simulink model "Refined_Model_38"  (R2020b)
settings: Solver=FixedStepAuto  StartTime=0.0  StopTime=500  FixedStep=0.1  RelTol=1e-3
values from neighbouring files (symbols this model uses):
  CovDist = RoadProfile(:,4)    [ICE_Val.m]
  Cx = VehicleDefine(7,3)    [BEV_Basictest.m]    (also in GPS_val.m; ICEBEV_Script.m; ICEBEV_Script_VECTO.m; ICE_Script.m)
  Dist = 1:length(MaxSpeedProfile)    [GPS_val.m]    (also in ICE_Script.m; ICE_Val.m = [1:CovDist(end)])
  DynRolRad = VehicleDefine(5,3)    [BEV_Basictest.m]    (also in GPS_val.m; ICEBEV_Script.m; ICEBEV_Script_VECTO.m; ICE_Script.m)
  EngineRpm = round(IntpTorCur(:,1))    [GPS_val.m]    (also in ICEBEV_Script.m; ICEBEV_Script_VECTO.m; ICE_Script.m; ICE_Script_SSVal.m)
  etaClutch = VehicleDefine(23,3)    [GPS_val.m]    (also in ICEBEV_Script.m; ICEBEV_Script_VECTO.m; ICE_Script.m; ICE_Script_SSVal.m)
  FCTableVal = FCMap(2:end,2:end)    [GPS_val.m]    (also in ICEBEV_Script.m; ICEBEV_Script_VECTO.m; ICE_Script.m; ICE_Script_SSVal.m)
  FDR = VehicleDefine(20,3)    [BEV_Basictest.m]    (also in GPS_val.m = VehicleDefine(22,3); ICEBEV_Script.m = VehicleDefine(22,3); ICEBEV_Script_VECTO.m = VehicleDefine(22,3); ICE_Script.m = VehicleDefine(22,3))
  Fr = VehicleDefine(13,3)    [BEV_Basictest.m]    (also in GPS_val.m; ICEBEV_Script.m; ICEBEV_Script_VECTO.m; ICE_Script.m)
  g = VehicleDefine(14,3)    [BEV_Basictest.m]    (also in GPS_val.m; ICEBEV_Script.m; ICEBEV_Script_VECTO.m; ICE_Script.m)
  GNo = GBXDefine(:,1)    [GPS_val.m]    (also in ICEBEV_Script.m; ICEBEV_Script_VECTO.m; ICE_Script.m; ICE_Script_SSVal.m)
  GRa = GBXDefine(:,2)    [GPS_val.m]    (also in ICEBEV_Script.m; ICEBEV_Script_VECTO.m; ICE_Script.m; ICE_Script_SSVal.m)
  InitVel = VehicleDefine(21,3)    [BEV_Basictest.m]    (also in GPS_val.m = VehicleDefine(24,3); ICEBEV_Script.m = VehicleDefine(24,3); ICEBEV_Script_VECTO.m = VehicleDefine(24,3); ICE_Script.m = VehicleDefine(24,3))
  IntpSlope = round(IntpSlope,1)    [GPS_val.m]    (also in ICE_Script.m; ICE_Val.m = A)
  Je = VehicleDefine(25,3)    [GPS_val.m]    (also in ICEBEV_Script.m; ICEBEV_Script_VECTO.m; ICE_Script.m; ICE_Script_SSVal.m)
  Jk = VehicleDefine(15,3)    [BEV_Basictest.m]    (also in GPS_val.m; ICEBEV_Script.m; ICEBEV_Script_VECTO.m; ICE_Script.m)
  Jm = VehicleDefine(16,3)    [GPS_val.m]    (also in ICEBEV_Script.m; ICEBEV_Script_VECTO.m; ICE_Script.m; ICE_Script_SSVal.m)
  MaxAcc = 1    [BEV_Basictest.m]    (also in GPS_val.m; ICEBEV_Script.m; ICEBEV_Script_VECTO.m; ICE_Script.m)
  MaxDec = 1    [BEV_Basictest.m]    (also in GPS_val.m; ICEBEV_Script.m; ICEBEV_Script_VECTO.m; ICE_Script.m)
  MaxSpeedProfile = FMSP    [GPS_val.m]    (also in ICE_Script.m; ICE_Val.m = repelem(SegSPLatinmps,SegLeninm))
  MaxTorValThrot = max(ThrotTableVal,[],2)    [GPS_val.m]    (also in ICEBEV_Script.m; ICEBEV_Script_VECTO.m; ICE_Script.m; ICE_Script_SSVal.m)
  Me = VehicleDefine(10,3)    [BEV_Basictest.m]    (also in GPS_val.m; ICEBEV_Script.m; ICEBEV_Script_VECTO.m; ICE_Script.m)
  MotoringTor = IntpTorCur(:,3)    [GPS_val.m]    (also in ICEBEV_Script.m; ICEBEV_Script_VECTO.m; ICE_Script.m; ICE_Script_SSVal.m)
  Mt = VehicleDefine(12,3)    [BEV_Basictest.m]    (also in GPS_val.m; ICEBEV_Script.m; ICEBEV_Script_VECTO.m; ICE_Script.m)
  Mtot = Mv+Me+Mt    [BEV_Basictest.m]    (also in GPS_val.m; ICEBEV_Script.m; ICEBEV_Script_VECTO.m; ICE_Script.m)
  Mv = VehicleDefine(9,3)    [BEV_Basictest.m]    (also in GPS_val.m; ICEBEV_Script.m; ICEBEV_Script_VECTO.m; ICE_Script.m)
  NoSteps = round(Dist(end))    [GPS_val.m]    (also in ICE_Script.m; ICE_Val.m = 3002)
  NoWhlFA = VehicleDefine(2,3)    [BEV_Basictest.m]    (also in GPS_val.m; ICE_Script.m; ICE_Val.m; ICE_Val_new.m)
  NoWhlRA = VehicleDefine(4,3)    [BEV_Basictest.m]    (also in GPS_val.m; ICE_Script.m; ICE_Val.m; ICE_Val_new.m)
  rho = VehicleDefine(6,3)    [BEV_Basictest.m]    (also in GPS_val.m; ICEBEV_Script.m; ICEBEV_Script_VECTO.m; ICE_Script.m)
  RpmBrkPnt = ThrottleMap(1,:)    [GPS_val.m]    (also in ICEBEV_Script.m; ICEBEV_Script_VECTO.m; ICE_Script.m; ICE_Script_SSVal.m)
  s = divisors(length(MaxSpeedProfile))    [GPS_val.m]    (also in ICEBEV_Script.m = round(FLoadTor); ICEBEV_Script_VECTO.m = round(FLoadTor); ICE_Script.m = round(FLoadTor); ICE_Script_SSVal.m = round(FLoadTor))
  SegNo = RoadProfile(:,1)    [ICE_Val.m]
  SegSPLatinmps = (sqrt(aMaxLat*g*CurRadinm))    [GPS_val.m]    (also in ICE_Script.m; ICE_Val.m)
  Sx = VehicleDefine(8,3)    [BEV_Basictest.m]    (also in GPS_val.m; ICEBEV_Script.m; ICEBEV_Script_VECTO.m; ICE_Script.m)
  ThrotPos = ThrotPos'    [GPS_val.m]    (also in ICEBEV_Script.m; ICEBEV_Script_VECTO.m; ICE_Script.m; ICE_Script_SSVal.m)
  ThrotTableVal = ThrottleMap(2:end,2:end)    [GPS_val.m]    (also in ICEBEV_Script.m; ICEBEV_Script_VECTO.m; ICE_Script.m; ICE_Script_SSVal.m)
undefined symbols (not defined in the file or in its folder): G1Inprpm, GInprpm, GInpTor, GTorLoss, MaxSpinG, MaxWhlTorinG, Stoptimes
libraries: simulink x3, autolibshared x1
settings Model: Creator=Kshitij  LastModifiedBy=Kshitij
settings DebuggingCC: AlgebraicLoopMsg=none

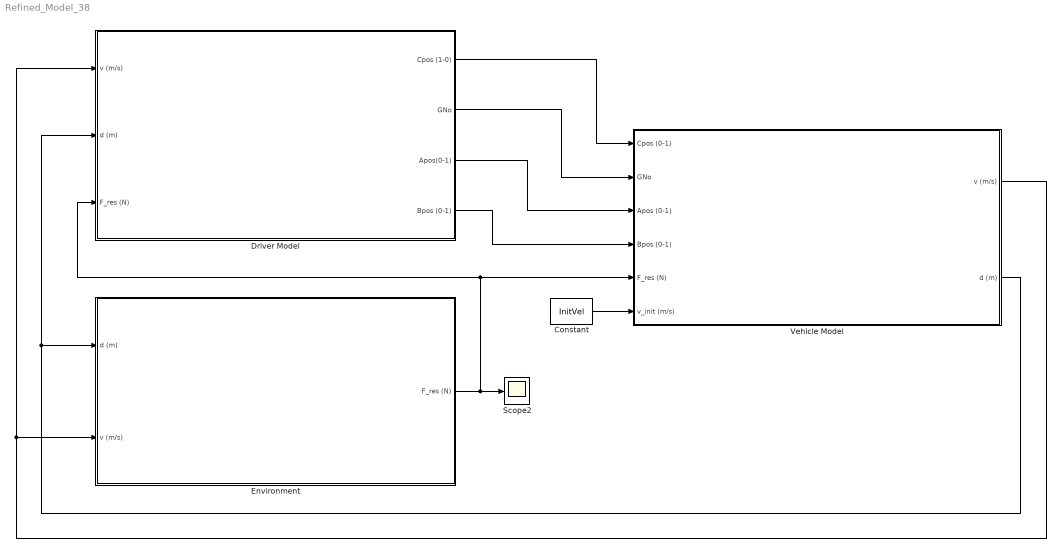
== system Refined_Model_38 ==
  Constant : Constant  Value=InitVel
  Driver Model : Subsystem
  Environment : Subsystem
  Scope2 : Scope
  Vehicle Model : Subsystem
  wires:
  Environment/1(F_res (N)) -> Driver Model/3(F_res (N)), Vehicle Model/5(F_res (N)), Scope2/1
  Vehicle Model/2(d (m)) -> Driver Model/2(d (m)), Environment/1(d (m))
  Vehicle Model/1(v (m/s)) -> Driver Model/1(v (m/s)), Environment/2(v (m/s))
  Constant/1 -> Vehicle Model/6(v_init (m/s))
  Driver Model/1(Cpos (1-0)) -> Vehicle Model/1(Cpos (0-1))
  Driver Model/2(GNo) -> Vehicle Model/2(GNo)
  Driver Model/3(Apos(0-1)) -> Vehicle Model/3(Apos (0-1))
  Driver Model/4(Bpos (0-1)) -> Vehicle Model/4(Bpos (0-1))

== system Refined_Model_38/Driver Model ==
  v (m/s) : Inport
  d (m) : Inport  Port=2
  F_res (N) : Inport  Port=3
  Acc/Dec Control : Subsystem
  Driver Throttle : Subsystem
  Gear and Clutch Definition : Subsystem
  Scope1 : Scope  NumInputPorts=2
  Cpos (1-0) : Outport
  GNo : Outport  Port=2
  Apos(0-1) : Outport  Port=3
  Bpos (0-1) : Outport  Port=4
  wires:
  Acc/Dec Control/2(Bpos (0-1)) -> Bpos (0-1)/1, Scope1/2  "Bpos (0-1)"
  d (m)/1 -> Acc/Dec Control/2(d (m))
  Gear and Clutch Definition/1(Cpos) -> Cpos (1-0)/1
  v (m/s)/1 -> Gear and Clutch Definition/2(v (m/s)), Acc/Dec Control/1(v (m/s))
  Gear and Clutch Definition/2(GNo) -> GNo/1, Driver Throttle/1(GNo)
  Driver Throttle/2(Apos (0-1)) -> Scope1/1, Apos(0-1)/1  "Apos(0-1)"
  Driver Throttle/1(T_w_req (Nm)) -> Gear and Clutch Definition/1(T_w_req (Nm))  "T_w_req (Nm)"
  F_res (N)/1 -> Driver Throttle/2(F_res (N))
  Acc/Dec Control/1(Apos(m/s^2)) -> Driver Throttle/3(Apos(m/s^2))

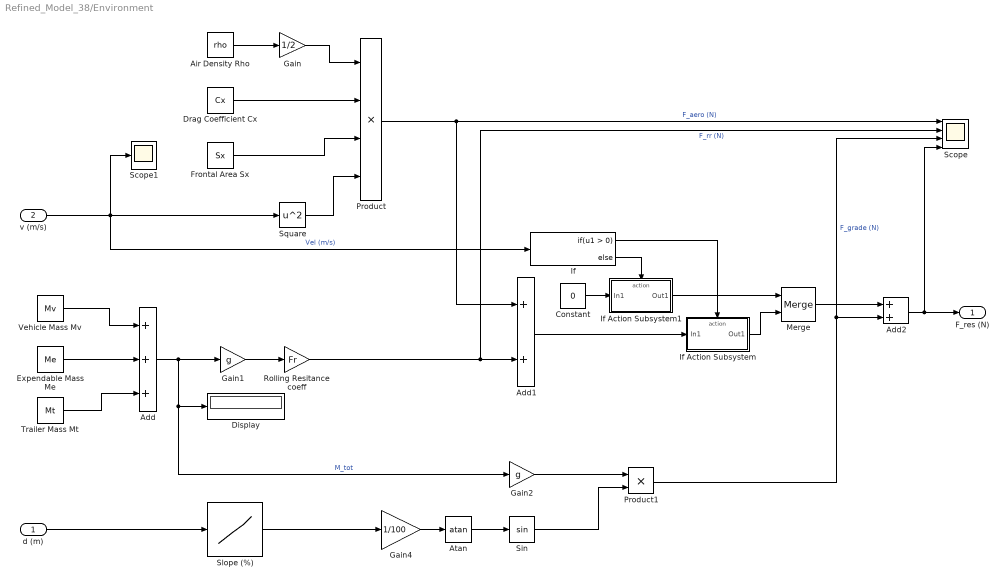
== system Refined_Model_38/Environment ==
  d (m) : Inport
  v (m/s) : Inport  Port=2
  Add : Sum  Inputs=+++
  Add1 : Sum
  Add2 : Sum
  Air Density Rho : Constant  Value=rho
  Atan : Trigonometry  Operator=atan
  Constant : Constant  Value=0
  Display : Display
  Drag Coefficient Cx : Constant  Value=Cx
  Expendable Mass Me : Constant  Value=Me
  Frontal Area Sx : Constant  Value=Sx
  Gain : Gain  Gain=1/2
  Gain1 : Gain  Gain=g
  Gain2 : Gain  Gain=g
  Gain4 : Gain  Gain=1/100
  If : If
  If Action Subsystem : Subsystem  TreatAsAtomicUnit=on
  If Action Subsystem1 : Subsystem  TreatAsAtomicUnit=on
  Merge : Merge
  Product : Product  Inputs=4
  Product1 : Product
  Rolling Resitance coeff : Gain  Gain=Fr
  Scope : Scope  NumInputPorts=4
  Scope1 : Scope
  Sin : Trigonometry
  Slope (%) : Lookup_n-D  NumberOfTableDimensions=1  BreakpointsForDimension1=Dist  Table=IntpSlope  InternalRulePriority=Speed  RndMeth=Simplest  InputSameDT=on
  Square : Math  Operator=square  SaturateOnIntegerOverflow=on
  Trailer Mass Mt : Constant  Value=Mt
  Vehicle Mass Mv : Constant  Value=Mv
  F_res (N) : Outport
  wires:
  Expendable Mass Me/1 -> Add/2
  Add/1 -> Display/1, Gain2/1, Gain1/1  "M_tot"
  Gain/1 -> Product/1
  Sin/1 -> Product1/2
  Product1/1 -> Scope/3, Add2/2  "F_grade (N)"
  Air Density Rho/1 -> Gain/1
  Drag Coefficient Cx/1 -> Product/2
  v (m/s)/1 -> Scope1/1, Square/1, If/1  "Vel (m/s)"
  d (m)/1 -> Slope (%)/1
  Gain2/1 -> Product1/1
  Trailer Mass Mt/1 -> Add/3
  Rolling Resitance coeff/1 -> Scope/2, Add1/2  "F_rr (N)"
  Square/1 -> Product/4
  Gain1/1 -> Rolling Resitance coeff/1
  Vehicle Mass Mv/1 -> Add/1
  Product/1 -> Scope/1, Add1/1  "F_aero (N)"
  Frontal Area Sx/1 -> Product/3
  If/1 -> If Action Subsystem/Action
  If/2 -> If Action Subsystem1/Action
  If Action Subsystem1/1(Out1) -> Merge/1
  Add1/1 -> If Action Subsystem/1(In1)
  If Action Subsystem/1(Out1) -> Merge/2
  Constant/1 -> If Action Subsystem1/1(In1)
  Merge/1 -> Add2/1
  Add2/1 -> F_res (N)/1, Scope/4
  Slope (%)/1 -> Gain4/1
  Atan/1 -> Sin/1
  Gain4/1 -> Atan/1

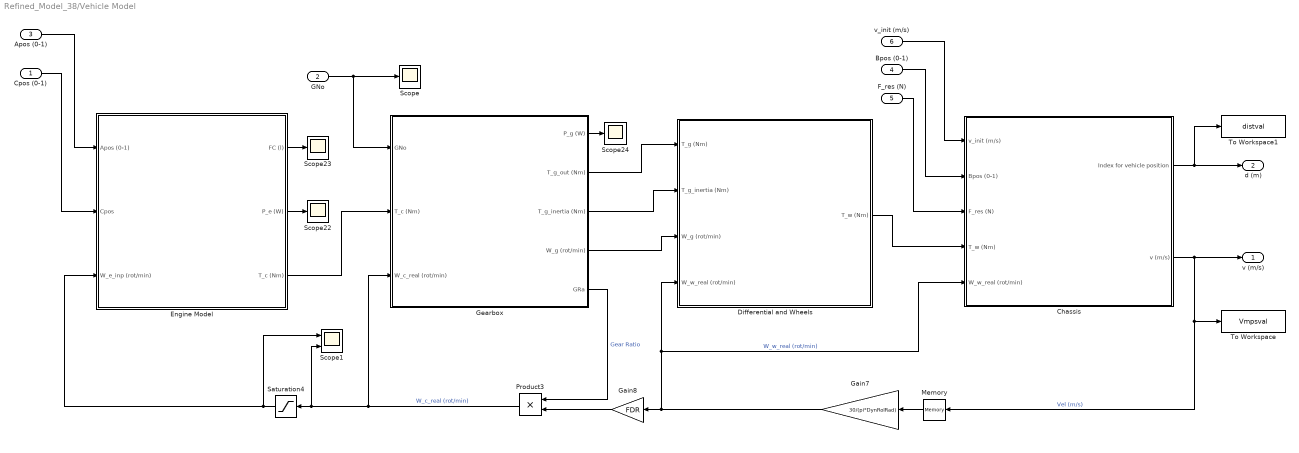
== system Refined_Model_38/Vehicle Model ==
  Cpos (0-1) : Inport
  GNo : Inport  Port=2
  Apos (0-1) : Inport  Port=3
  Bpos (0-1) : Inport  Port=4
  F_res (N) : Inport  Port=5
  v_init (m/s) : Inport  Port=6
  Chassis : Subsystem
  Differential and Wheels : Subsystem
  Engine Model : Subsystem
  Gain7 : Gain  Gain=30/(pi*DynRolRad)
  Gain8 : Gain  Gain=FDR
  Gearbox : Subsystem
  Memory : Memory
  Product3 : Product
  Saturation4 : Saturate  UpperLimit=max(EngineRpm)  LowerLimit=min(EngineRpm)
  Scope{,22..24} (4 alike) : Scope
  Scope1 : Scope  NumInputPorts=2
  To Workspace : ToWorkspace  VariableName=Vmpsval  SaveFormat=Timeseries  SampleTime=-1
  To Workspace1 : ToWorkspace  VariableName=distval  SaveFormat=Timeseries  SampleTime=-1
  v (m/s) : Outport
  d (m) : Outport  Port=2
  wires:
  Gearbox/2(T_g_out (Nm)) -> Differential and Wheels/1(T_g (Nm))
  Gearbox/4(W_g (rot/min)) -> Differential and Wheels/3(W_g (rot/min))
  Gearbox/3(T_g_inertia (Nm)) -> Differential and Wheels/2(T_g_inertia (Nm))
  Chassis/1(Index for vehicle position) -> To Workspace1/1, d (m)/1
  Bpos (0-1)/1 -> Chassis/2(Bpos (0-1))
  v_init (m/s)/1 -> Chassis/1(v_init (m/s))
  Differential and Wheels/1(T_w (Nm)) -> Chassis/4(T_w (Nm))
  F_res (N)/1 -> Chassis/3(F_res (N))
  Gearbox/1(P_g (W)) -> Scope24/1
  Engine Model/3(T_c (Nm)) -> Gearbox/2(T_c (Nm))
  Apos (0-1)/1 -> Engine Model/1(Apos (0-1))
  Engine Model/2(P_e (W)) -> Scope22/1
  Engine Model/1(FC (l)) -> Scope23/1
  GNo/1 -> Gearbox/1(GNo), Scope/1
  Chassis/2(v (m/s)) -> v (m/s)/1, Memory/1, To Workspace/1  "Vel (m/s)"
  Gearbox/5(GRa) -> Product3/1  "Gear Ratio"
  Gain8/1 -> Product3/2
  Gain7/1 -> Gain8/1, Chassis/5(W_w_real (rot/min)), Differential and Wheels/4(W_w_real (rot/min))  "W_w_real (rot/min)"
  Cpos (0-1)/1 -> Engine Model/2(Cpos)
  Product3/1 -> Scope1/2, Saturation4/1, Gearbox/3(W_c_real (rot/min))  "W_c_real (rot/min)"
  Saturation4/1 -> Scope1/1, Engine Model/3(W_e_inp (rot/min))
  Memory/1 -> Gain7/1

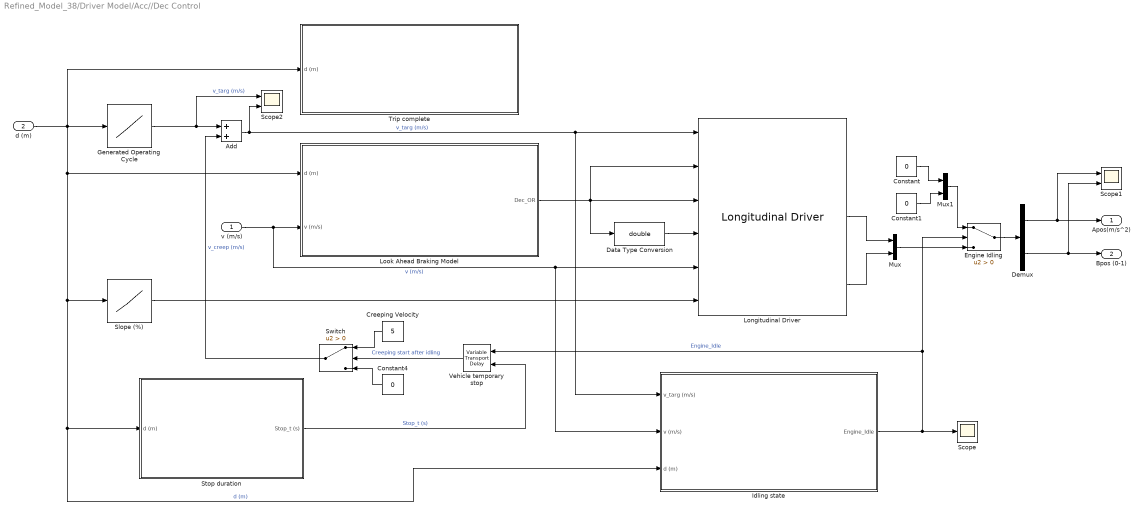
== system Refined_Model_38/Driver Model/Acc//Dec Control ==
  v (m/s) : Inport
  d (m) : Inport  Port=2
  Add : Sum
  Constant : Constant  Value=0
  Constant1 : Constant  Value=0
  Constant4 : Constant  Value=0
  Creeping Velocity : Constant  Value=5
  Data Type Conversion : DataTypeConversion  OutDataTypeStr=double
  Demux : Demux  Outputs=2
  Engine Idling : Switch  Criteria=u2 > Threshold
  Generated Operating Cycle : Lookup_n-D  NumberOfTableDimensions=1  BreakpointsForDimension1=Dist  BreakpointsForDimension2=G1Inprpm  Table=MaxSpeedProfile  InterpMethod=Linear Lagrange  InternalRulePriority=Speed  RndMeth=Simplest  InputSameDT=on
  Idling state : Subsystem
  Longitudinal Driver : autolibshared/Longitudinal Driver  extAccelOvr=off  extDecelOvr=on  extAccelHld=off  extDecelHld=off  extAccelZero=on  extDecelZero=off  cntrlType=PI  shftType=None  velUnits=m/s  gearOut=off  Kp=150  Ki=1000  Kff=0  Kg=0  VehVelVec=[0 100]  KffVec=[.1 .1]  KpVec=[10 10]  KiVec=[5 5]  KgVec=[0 0]  m=1500  Kpt=3000  tau=.1  L=2  aR=200  bR=2.5  cR=.5  g=9.81  vnom=100  Kaw=0  tauerr=0  tauPt=2  GearInit=0  tShift=.1  pdlVec=[0.1 0.4 0.5 0.9]  upShftTbl=[-1 12.9375 26.4375 39.9375 51.18749999999999 62.4375 72.84375 83.25;-1 16.3125 29.8125 43.3125 54.5624 65.8125 76.78125 87.75;-1 19.6875 33.1875 46.68749999999999 57.9375 69.1875 80.71875 92.25;-1 33 52.5 77.25 100.5 138.75 161.875 185]  dwnShftTbl=[1 9.5625 23.0625 36.5625 47.8125 59.0625 68.90625 78.75;1 12.9375 26.4375 39.9375 51.18749999999999 62.4375 72.84375 83.25;1 16.3125 29.8125 43.3125 54.562499 65.8125 76.78125 87.75;1 19.6875 33.1875 46.68749999999999 57.9375 69.1875 80.71875 92.25]  tClutch=.5  tRev=.5  tPark=120  aMode=1  UpGearVec="[0  1  2  3  4  5  6  7]"  DownGearVec="[1  2  3  4  5  6  7  8]"
      settings: SourceProductBaseCode=PW,MT,UV,VE,VP
  Look Ahead Braking Model : Subsystem
  Mux : Mux  Inputs=2
  Mux1 : Mux  Inputs=2
  Scope : Scope
  Scope1 : Scope  NumInputPorts=2
  Scope2 : Scope  NumInputPorts=2
  Slope (%) : Lookup_n-D  NumberOfTableDimensions=1  BreakpointsForDimension1=Dist  Table=IntpSlope  InternalRulePriority=Speed  RndMeth=Simplest  InputSameDT=on
  Stop duration : Subsystem
  Switch : Switch  Criteria=u2 > Threshold
  Trip complete : Subsystem
  Vehicle temporary stop : VariableTransportDelay  VariableDelayType=Variable transport delay  MaximumDelay=10
  Apos(m/s^2) : Outport
  Bpos (0-1) : Outport  Port=2
  wires:
  Add/1 -> Scope2/2, Idling state/1(v_targ (m/s)), Longitudinal Driver/1  "v_targ (m/s)"
  Slope (%)/1 -> Longitudinal Driver/6
  Longitudinal Driver/2 -> Mux/1
  Look Ahead Braking Model/1(Dec_OR) -> Longitudinal Driver/2, Longitudinal Driver/3, Data Type Conversion/1
  Demux/1 -> Scope1/1, Apos(m/s^2)/1
  Demux/2 -> Scope1/2, Bpos (0-1)/1
  Constant/1 -> Mux1/1
  Mux/1 -> Engine Idling/3
  Constant1/1 -> Mux1/2
  Mux1/1 -> Engine Idling/1
  Engine Idling/1 -> Demux/1
  d (m)/1 -> Idling state/3(d (m)), Stop duration/1(d (m)), Slope (%)/1, Look Ahead Braking Model/1(d (m)), Trip complete/1(d (m)), Generated Operating Cycle/1  "d (m)"
  v (m/s)/1 -> Longitudinal Driver/5, Idling state/2(v (m/s)), Look Ahead Braking Model/2(v (m/s))  "v (m/s)"
  Generated Operating Cycle/1 -> Scope2/1, Add/1  "v_targ (m/s)"
  Vehicle temporary stop/1 -> Switch/2  "Creeping start after idling"
  Switch/1 -> Add/2  "v_creep (m/s)"
  Constant4/1 -> Switch/3
  Creeping Velocity/1 -> Switch/1
  Idling state/1(Engine_Idle) -> Scope/1, Engine Idling/2, Vehicle temporary stop/1  "Engine_Idle"
  Stop duration/1(Stop_t (s)) -> Vehicle temporary stop/2  "Stop_t (s)"
  Data Type Conversion/1 -> Longitudinal Driver/4
  Longitudinal Driver/3 -> Mux/2

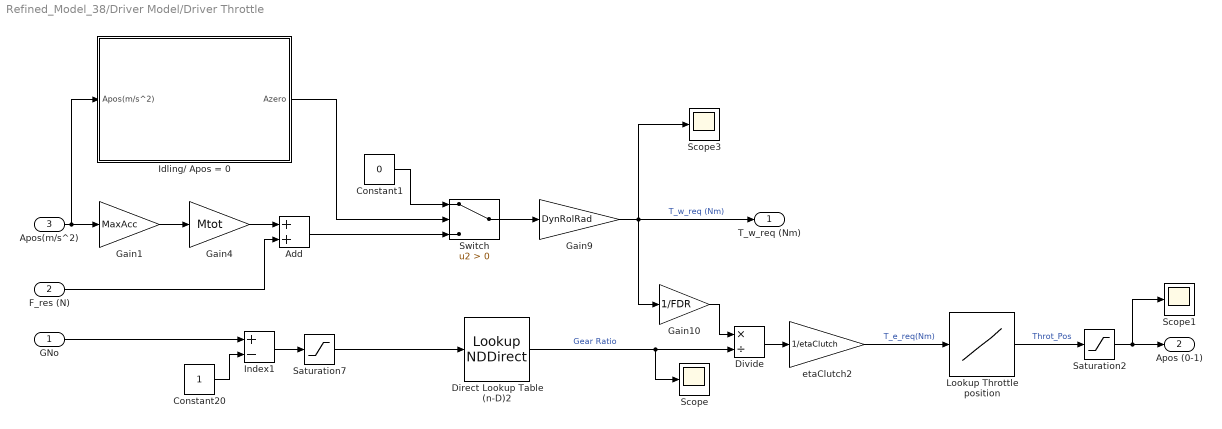
== system Refined_Model_38/Driver Model/Driver Throttle ==
  GNo : Inport
  F_res (N) : Inport  Port=2
  Apos(m/s^2) : Inport  Port=3
  Add : Sum
  Constant1 : Constant  Value=0
  Constant20 : Constant
  Direct Lookup Table (n-D)2 : LookupNDDirect  NumberOfTableDimensions=1  Table=GRa
  Divide : Product  Inputs=*/
  Gain1 : Gain  Gain=MaxAcc
  Gain10 : Gain  Gain=1/FDR
  Gain4 : Gain  Gain=Mtot
  Gain9 : Gain  Gain=DynRolRad
  Idling/ Apos = 0 : Subsystem
  Index1 : Sum  Inputs=+-
  Lookup Throttle position : Lookup_n-D  NumberOfTableDimensions=1  BreakpointsForDimension1=MaxTorValThrot  Table=ThrotPos  InternalRulePriority=Speed  RndMeth=Simplest  InputSameDT=on
  Saturation2 : Saturate  UpperLimit=1  LowerLimit=0
  Saturation7 : Saturate  UpperLimit=inf  LowerLimit=0
  Scope : Scope
  Scope1 : Scope
  Scope3 : Scope
  Switch : Switch  Criteria=u2 > Threshold
  etaClutch2 : Gain  Gain=1/etaClutch
  T_w_req (Nm) : Outport
  Apos (0-1) : Outport  Port=2
  wires:
  etaClutch2/1 -> Lookup Throttle position/1  "T_e_req(Nm)"
  Add/1 -> Switch/3
  Gain9/1 -> Scope3/1, T_w_req (Nm)/1, Gain10/1  "T_w_req (Nm)"
  Gain10/1 -> Divide/1
  Gain4/1 -> Add/1
  Divide/1 -> etaClutch2/1
  F_res (N)/1 -> Add/2
  Lookup Throttle position/1 -> Saturation2/1  "Throt_Pos"
  Saturation2/1 -> Apos (0-1)/1, Scope1/1
  Apos(m/s^2)/1 -> Idling/ Apos = 0/1(Apos(m/s^2)), Gain1/1
  Gain1/1 -> Gain4/1
  Constant20/1 -> Index1/2
  GNo/1 -> Index1/1
  Index1/1 -> Saturation7/1
  Saturation7/1 -> Direct Lookup Table (n-D)2/1
  Direct Lookup Table (n-D)2/1 -> Scope/1, Divide/2  "Gear Ratio"
  Switch/1 -> Gain9/1
  Constant1/1 -> Switch/1
  Idling/ Apos = 0/1(Azero) -> Switch/2

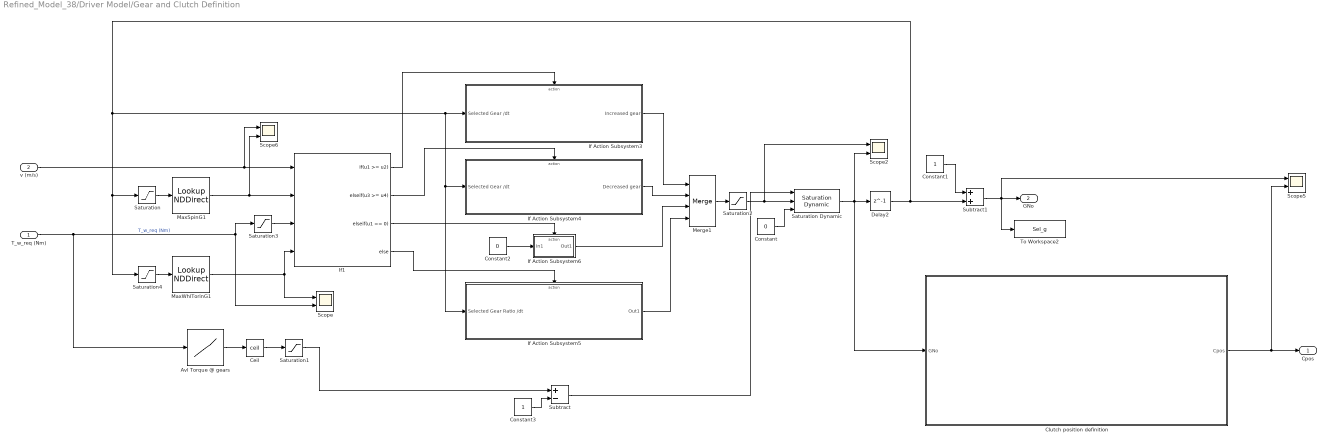
== system Refined_Model_38/Driver Model/Gear and Clutch Definition ==
  T_w_req (Nm) : Inport
  v (m/s) : Inport  Port=2
  Avl Torque @ gears : Lookup_n-D  NumberOfTableDimensions=1  BreakpointsForDimension1=flip(MaxWhlTorinG)  Table=flip(GNo)  InternalRulePriority=Speed  RndMeth=Simplest  InputSameDT=on
  Ceil : Rounding  Operator=ceil
  Clutch position definition : Subsystem
  Constant : Constant  Value=0
  Constant1 : Constant
  Constant2 : Constant  Value=0
  Constant3 : Constant
  Delay2 : Delay  DelayLength=1
  If Action Subsystem3 : Subsystem  TreatAsAtomicUnit=on
  If Action Subsystem4 : Subsystem  TreatAsAtomicUnit=on
  If Action Subsystem5 : Subsystem  TreatAsAtomicUnit=on
  If Action Subsystem6 : Subsystem  TreatAsAtomicUnit=on
  If1 : If  NumInputs=4  IfExpression=u1 >= u2  ElseIfExpressions=u3 >= u4,u1 == 0
  MaxSpinG1 : LookupNDDirect  NumberOfTableDimensions=1  Table=MaxSpinG
  MaxWhlTorinG1 : LookupNDDirect  NumberOfTableDimensions=1  Table=MaxWhlTorinG
  Merge1 : Merge  Inputs=4
  Saturation : Saturate  UpperLimit=inf  LowerLimit=0
  Saturation Dynamic : simulink/Discontinuities/Saturation Dynamic  OutMin=[]  OutMax=[]  OutDataTypeStr=Inherit: Same as second input  OutDataType=fixdt(1, 16)  OutScaling=2^-10  DoSatur=off
  Saturation1 : Saturate  UpperLimit=max(GNo)  LowerLimit=0
  Saturation2 : Saturate  UpperLimit=max(GNo)-1  LowerLimit=0
  Saturation3 : Saturate  UpperLimit=inf  LowerLimit=0
  Saturation4 : Saturate  UpperLimit=inf  LowerLimit=0
  Scope{,2,5..6} (4 alike) : Scope  NumInputPorts=2
  Subtract : Sum  Inputs=+-
  Subtract1 : Sum
  To Workspace2 : ToWorkspace  VariableName=Sel_g  SaveFormat=Timeseries  SampleTime=-1
  Cpos : Outport
  GNo : Outport  Port=2
  wires:
  Clutch position definition/1(Cpos) -> Scope5/2, Cpos/1
  If1/2 -> If Action Subsystem4/Action
  If Action Subsystem4/1(Decreased gear) -> Merge1/2
  If1/4 -> If Action Subsystem5/Action
  If Action Subsystem3/1(Increased gear) -> Merge1/1
  MaxSpinG1/1 -> Scope6/2, If1/2
  If Action Subsystem5/1(Out1) -> Merge1/4
  MaxWhlTorinG1/1 -> Scope/1, If1/4
  If1/1 -> If Action Subsystem3/Action
  Saturation3/1 -> If1/3
  T_w_req (Nm)/1 -> Saturation3/1, Scope/2, Avl Torque @ gears/1  "T_w_req (Nm)"
  Constant1/1 -> Subtract1/1
  Saturation/1 -> MaxSpinG1/1
  Saturation4/1 -> MaxWhlTorinG1/1
  Delay2/1 -> Subtract1/2, If Action Subsystem3/1(Selected Gear /dt), If Action Subsystem5/1(Selected Gear Ratio /dt), If Action Subsystem4/1(Selected Gear /dt), Saturation/1, Saturation4/1
  Subtract1/1 -> Scope5/1, GNo/1, To Workspace2/1
  v (m/s)/1 -> Scope6/1, If1/1
  If1/3 -> If Action Subsystem6/Action
  Constant2/1 -> If Action Subsystem6/1(In1)
  If Action Subsystem6/1(Out1) -> Merge1/3
  Merge1/1 -> Saturation2/1
  Avl Torque @ gears/1 -> Ceil/1
  Ceil/1 -> Saturation1/1
  Saturation Dynamic/1 -> Scope2/2, Clutch position definition/1(GNo), Delay2/1
  Subtract/1 -> Saturation Dynamic/1
  Constant3/1 -> Subtract/2
  Saturation1/1 -> Subtract/1
  Saturation2/1 -> Scope2/1, Saturation Dynamic/2
  Constant/1 -> Saturation Dynamic/3

== system Refined_Model_38/Environment/If Action Subsystem ==
  In1 : Inport
  Action Port : ActionPort  ActionPortLabel=if(u1 > 0)
  Out1 : Outport
  wires:
  In1/1 -> Out1/1

== system Refined_Model_38/Environment/If Action Subsystem1 ==
  In1 : Inport
  Action Port : ActionPort  ActionPortLabel=else
  Out1 : Outport
  wires:
  In1/1 -> Out1/1

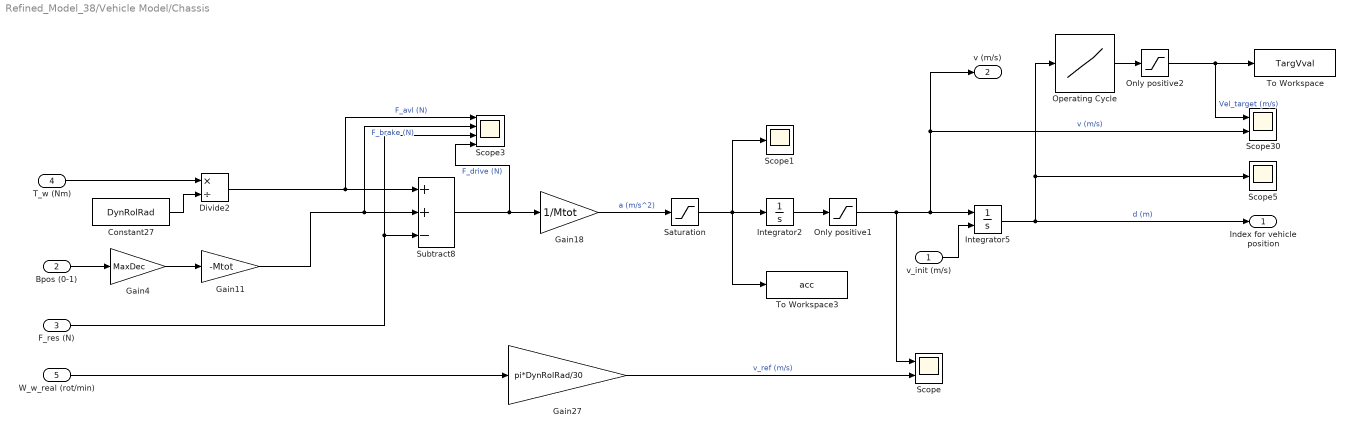
== system Refined_Model_38/Vehicle Model/Chassis ==
  v_init (m/s) : Inport
  Bpos (0-1) : Inport  Port=2
  F_res (N) : Inport  Port=3
  T_w (Nm) : Inport  Port=4
  W_w_real (rot/min) : Inport  Port=5
  Constant27 : Constant  Value=DynRolRad
  Divide2 : Product  Inputs=*/
  Gain11 : Gain  Gain=-Mtot
  Gain18 : Gain  Gain=1/Mtot
  Gain27 : Gain  Gain=pi*DynRolRad/30
  Gain4 : Gain  Gain=MaxDec
  Integrator2 : Integrator  ContinuousStateAttributes='acceleration'
  Integrator5 : Integrator  InitialConditionSource=external  ContinuousStateAttributes='velocity'
  Only positive1 : Saturate  UpperLimit=inf  LowerLimit=0
  Only positive2 : Saturate  UpperLimit=inf  LowerLimit=0
  Operating Cycle : Lookup_n-D  NumberOfTableDimensions=1  BreakpointsForDimension1=Dist  BreakpointsForDimension2=G1Inprpm  Table=MaxSpeedProfile  InterpMethod=Linear Lagrange  InternalRulePriority=Speed  RndMeth=Simplest  InputSameDT=on
  Saturation : Saturate  UpperLimit=MaxAcc  LowerLimit=-(MaxDec)
  Scope : Scope  NumInputPorts=2
  Scope1 : Scope
  Scope3 : Scope  NumInputPorts=4
  Scope30 : Scope  NumInputPorts=2
  Scope5 : Scope
  Subtract8 : Sum  Inputs=++-
  To Workspace : ToWorkspace  VariableName=TargVval  SaveFormat=Timeseries  SampleTime=-1
  To Workspace3 : ToWorkspace  VariableName=acc  SaveFormat=Timeseries  SampleTime=-1
  Index for vehicle position : Outport
  v (m/s) : Outport  Port=2
  wires:
  Constant27/1 -> Divide2/2
  Subtract8/1 -> Scope3/4, Gain18/1  "F_drive (N)"
  Divide2/1 -> Subtract8/1, Scope3/1  "F_avl (N)"
  Integrator5/1 -> Index for vehicle position/1, Scope5/1, Operating Cycle/1  "d (m)"
  Integrator2/1 -> Only positive1/1
  T_w (Nm)/1 -> Divide2/1
  Gain11/1 -> Subtract8/2, Scope3/2  "F_brake (N)"
  Only positive1/1 -> Scope/1, v (m/s)/1, Scope30/2, Integrator5/1  "v (m/s)"
  v_init (m/s)/1 -> Integrator5/2
  Gain27/1 -> Scope/2  "v_ref (m/s)"
  Operating Cycle/1 -> Only positive2/1
  Gain18/1 -> Saturation/1  "a (m/s^2)"
  W_w_real (rot/min)/1 -> Gain27/1
  Bpos (0-1)/1 -> Gain4/1
  Gain4/1 -> Gain11/1
  F_res (N)/1 -> Subtract8/3, Scope3/3
  Saturation/1 -> Integrator2/1, To Workspace3/1, Scope1/1
  Only positive2/1 -> To Workspace/1, Scope30/1  "Vel_target (m/s)"

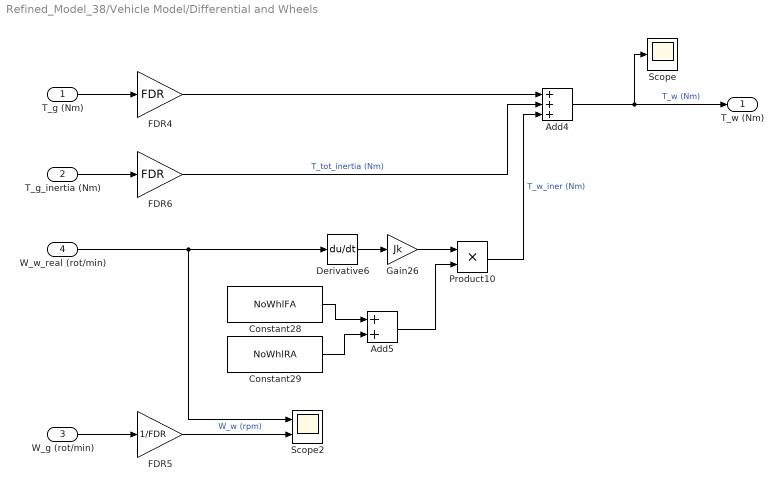
== system Refined_Model_38/Vehicle Model/Differential and Wheels ==
  T_g (Nm) : Inport
  T_g_inertia (Nm) : Inport  Port=2
  W_g (rot/min) : Inport  Port=3
  W_w_real (rot/min) : Inport  Port=4
  Add4 : Sum  Inputs=+++
  Add5 : Sum
  Constant28 : Constant  Value=NoWhlFA
  Constant29 : Constant  Value=NoWhlRA
  Derivative6 : Derivative
  FDR4 : Gain  Gain=FDR
  FDR5 : Gain  Gain=1/FDR
  FDR6 : Gain  Gain=FDR
  Gain26 : Gain  Gain=Jk
  Product10 : Product
  Scope : Scope
  Scope2 : Scope  NumInputPorts=2
  T_w (Nm) : Outport
  wires:
  Product10/1 -> Add4/3  "T_w_iner (Nm)"
  Derivative6/1 -> Gain26/1
  Add5/1 -> Product10/2
  Constant29/1 -> Add5/2
  FDR6/1 -> Add4/2  "T_tot_inertia (Nm)"
  Constant28/1 -> Add5/1
  FDR4/1 -> Add4/1
  FDR5/1 -> Scope2/2  "W_w (rpm)"
  Gain26/1 -> Product10/1
  T_g_inertia (Nm)/1 -> FDR6/1
  Add4/1 -> Scope/1, T_w (Nm)/1  "T_w (Nm)"
  T_g (Nm)/1 -> FDR4/1
  W_g (rot/min)/1 -> FDR5/1
  W_w_real (rot/min)/1 -> Scope2/1, Derivative6/1

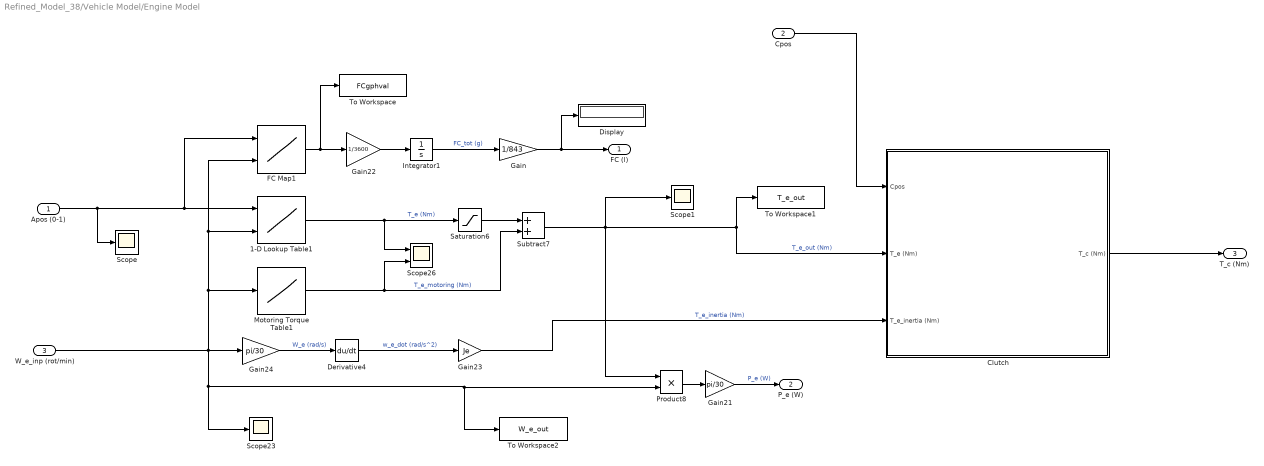
== system Refined_Model_38/Vehicle Model/Engine Model ==
  Apos (0-1) : Inport
  Cpos : Inport  Port=2
  W_e_inp (rot/min) : Inport  Port=3
  1-D Lookup Table1 : Lookup_n-D  BreakpointsForDimension1=ThrotPos  BreakpointsForDimension2=RpmBrkPnt  Table=ThrotTableVal  InternalRulePriority=Speed  RndMeth=Simplest  InputSameDT=on
      settings: InputPortMap=u0,u1
  Clutch : Subsystem
  Derivative4 : Derivative
  Display : Display
  FC Map1 : Lookup_n-D  BreakpointsForDimension1=ThrotPos  BreakpointsForDimension2=RpmBrkPnt  Table=FCTableVal  InternalRulePriority=Speed  RndMeth=Simplest  InputSameDT=on
      settings: InputPortMap=u0,u1
  Gain : Gain  Gain=1/843
  Gain21 : Gain  Gain=pi/30
  Gain22 : Gain  Gain=1/3600
  Gain23 : Gain  Gain=Je
  Gain24 : Gain  Gain=pi/30
  Integrator1 : Integrator
  Motoring Torque Table1 : Lookup_n-D  NumberOfTableDimensions=1  BreakpointsForDimension1=EngineRpm  BreakpointsForDimension2=G1Inprpm  Table=MotoringTor  InterpMethod=Linear Lagrange  InternalRulePriority=Speed  RndMeth=Simplest  InputSameDT=on
  Product8 : Product
  Saturation6 : Saturate  UpperLimit=inf  LowerLimit=0
  Scope : Scope
  Scope1 : Scope
  Scope23 : Scope
  Scope26 : Scope  NumInputPorts=2
  Subtract7 : Sum
  To Workspace : ToWorkspace  VariableName=FCgphval  SaveFormat=Timeseries  SampleTime=-1
  To Workspace1 : ToWorkspace  VariableName=T_e_out  SaveFormat=Timeseries  SampleTime=-1
  To Workspace2 : ToWorkspace  VariableName=W_e_out  SaveFormat=Timeseries  SampleTime=-1
  FC (l) : Outport
  P_e (W) : Outport  Port=2
  T_c (Nm) : Outport  Port=3
  wires:
  Motoring Torque Table1/1 -> Subtract7/2, Scope26/2  "T_e_motoring (Nm)"
  Integrator1/1 -> Gain/1  "FC_tot (g)"
  Derivative4/1 -> Gain23/1  "w_e_dot (rad/s^2)"
  W_e_inp (rot/min)/1 -> Scope23/1, To Workspace2/1, Product8/2, FC Map1/2, 1-D Lookup Table1/2, Motoring Torque Table1/1, Gain24/1
  Product8/1 -> Gain21/1
  Apos (0-1)/1 -> FC Map1/1, 1-D Lookup Table1/1, Scope/1
  1-D Lookup Table1/1 -> Saturation6/1, Scope26/1  "T_e (Nm)"
  Gain24/1 -> Derivative4/1  "W_e (rad/s)"
  Gain23/1 -> Clutch/3(T_e_inertia (Nm))  "T_e_inertia (Nm)"
  Gain21/1 -> P_e (W)/1  "P_e (W)"
  Gain22/1 -> Integrator1/1
  Subtract7/1 -> To Workspace1/1, Clutch/2(T_e (Nm)), Scope1/1, Product8/1  "T_e_out (Nm)"
  FC Map1/1 -> To Workspace/1, Gain22/1
  Saturation6/1 -> Subtract7/1
  Clutch/1(T_c (Nm)) -> T_c (Nm)/1
  Cpos/1 -> Clutch/1(Cpos)
  Gain/1 -> Display/1, FC (l)/1

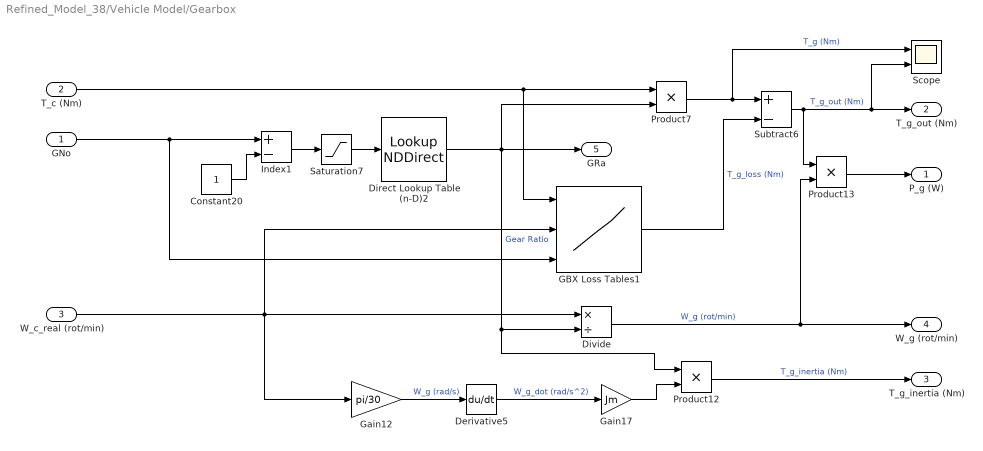
== system Refined_Model_38/Vehicle Model/Gearbox ==
  GNo : Inport
  T_c (Nm) : Inport  Port=2
  W_c_real (rot/min) : Inport  Port=3
  Constant20 : Constant
  Derivative5 : Derivative
  Direct Lookup Table (n-D)2 : LookupNDDirect  NumberOfTableDimensions=1  Table=GRa
  Divide : Product  Inputs=*/
  GBX Loss Tables1 : Lookup_n-D  NumberOfTableDimensions=3  BreakpointsForDimension1=GInpTor  BreakpointsForDimension2=GInprpm  BreakpointsForDimension3=GNo  Table=GTorLoss  InterpMethod=Linear Lagrange  InternalRulePriority=Speed  RndMeth=Simplest  InputSameDT=on
      settings: InputPortMap=u0,u1,u2
  Gain12 : Gain  Gain=pi/30
  Gain17 : Gain  Gain=Jm
  Index1 : Sum  Inputs=+-
  Product12 : Product
  Product13 : Product
  Product7 : Product
  Saturation7 : Saturate  UpperLimit=inf  LowerLimit=0
  Scope : Scope  NumInputPorts=2
  Subtract6 : Sum  Inputs=+-
  P_g (W) : Outport
  T_g_out (Nm) : Outport  Port=2
  T_g_inertia (Nm) : Outport  Port=3
  W_g (rot/min) : Outport  Port=4
  GRa : Outport  Port=5
  wires:
  Product12/1 -> T_g_inertia (Nm)/1  "T_g_inertia (Nm)"
  GNo/1 -> GBX Loss Tables1/3, Index1/1
  Gain17/1 -> Product12/2
  T_c (Nm)/1 -> GBX Loss Tables1/1, Product7/1
  Product7/1 -> Scope/1, Subtract6/1  "T_g (Nm)"
  Divide/1 -> W_g (rot/min)/1, Product13/2  "W_g (rot/min)"
  Subtract6/1 -> Scope/2, T_g_out (Nm)/1, Product13/1  "T_g_out (Nm)"
  Derivative5/1 -> Gain17/1  "W_g_dot (rad/s^2)"
  Direct Lookup Table (n-D)2/1 -> Product7/2, GRa/1, Product12/1, Divide/2  "Gear Ratio"
  Saturation7/1 -> Direct Lookup Table (n-D)2/1
  Gain12/1 -> Derivative5/1  "W_g (rad/s)"
  Constant20/1 -> Index1/2
  GBX Loss Tables1/1 -> Subtract6/2  "T_g_loss (Nm)"
  Index1/1 -> Saturation7/1
  Product13/1 -> P_g (W)/1
  W_c_real (rot/min)/1 -> GBX Loss Tables1/2, Gain12/1, Divide/1

== system Refined_Model_38/Driver Model/Acc//Dec Control/Idling state ==
  v_targ (m/s) : Inport
  v (m/s) : Inport  Port=2
  d (m) : Inport  Port=3
  Constant2 : Constant
  Constant3 : Constant  Value=0
  Delay : Delay  DelayLength=1
  Idling at stop point : If  NumInputs=3  IfExpression=u1 == 0 & u2 < 0 & u3 > 10
  If Action Subsystem : Subsystem  TreatAsAtomicUnit=on
  If Action Subsystem1 : Subsystem  TreatAsAtomicUnit=on
  Merge : Merge
  Subtract : Sum  Inputs=+-
  Engine_Idle : Outport
  wires:
  Subtract/1 -> Idling at stop point/2
  d (m)/1 -> Idling at stop point/3
  Constant2/1 -> If Action Subsystem/1(In1)
  If Action Subsystem/1(Out1) -> Merge/1
  Merge/1 -> Delay/1
  Idling at stop point/1 -> If Action Subsystem/Action
  Constant3/1 -> If Action Subsystem1/1(In1)
  v (m/s)/1 -> Subtract/2, Idling at stop point/1
  Idling at stop point/2 -> If Action Subsystem1/Action
  If Action Subsystem1/1(Out1) -> Merge/2
  Delay/1 -> Engine_Idle/1
  v_targ (m/s)/1 -> Subtract/1

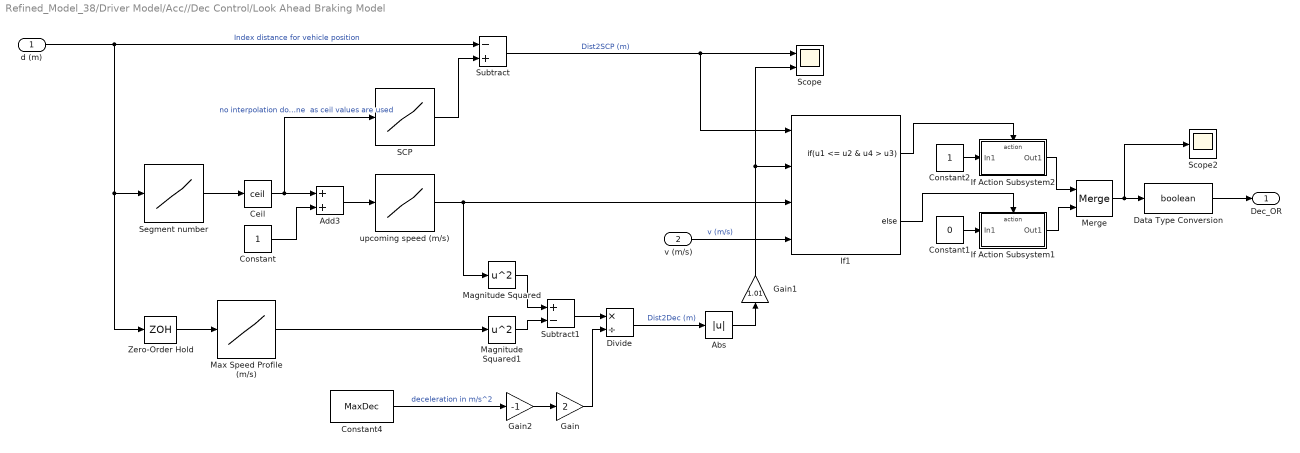
== system Refined_Model_38/Driver Model/Acc//Dec Control/Look Ahead Braking Model ==
  d (m) : Inport
  v (m/s) : Inport  Port=2
  Abs : Abs
  Add3 : Sum
  Ceil : Rounding  Operator=ceil
  Constant : Constant
  Constant1 : Constant  Value=0
  Constant2 : Constant
  Constant4 : Constant  Value=MaxDec
  Data Type Conversion : DataTypeConversion  OutDataTypeStr=boolean
  Divide : Product  Inputs=*/
  Gain : Gain  Gain=2
  Gain1 : Gain  Gain=1.01
  Gain2 : Gain  Gain=-1
  If Action Subsystem1 : Subsystem  TreatAsAtomicUnit=on
  If Action Subsystem2 : Subsystem  TreatAsAtomicUnit=on
  If1 : If  NumInputs=4  IfExpression=u1 <= u2 & u4 > u3
  Magnitude Squared : Math  Operator=square  SaturateOnIntegerOverflow=on
  Magnitude Squared1 : Math  Operator=square  SaturateOnIntegerOverflow=on
  Max Speed Profile (m/s) : Lookup_n-D  NumberOfTableDimensions=1  BreakpointsForDimension1=Dist  BreakpointsForDimension2=G1Inprpm  Table=MaxSpeedProfile  InterpMethod=Linear Lagrange  InternalRulePriority=Speed  RndMeth=Simplest  InputSameDT=on
  Merge : Merge
  SCP : Lookup_n-D  NumberOfTableDimensions=1  BreakpointsForDimension1=SegNo  BreakpointsForDimension2=G1Inprpm  Table=CovDist  InterpMethod=Linear Lagrange  InternalRulePriority=Speed  RndMeth=Simplest  InputSameDT=on
  Scope : Scope  NumInputPorts=2
  Scope2 : Scope
  Segment number : Lookup_n-D  NumberOfTableDimensions=1  BreakpointsForDimension1=CovDist  BreakpointsForDimension2=G1Inprpm  Table=SegNo  InterpMethod=Linear Lagrange  InternalRulePriority=Speed  RndMeth=Simplest  InputSameDT=on
  Subtract : Sum  Inputs=-+
  Subtract1 : Sum  Inputs=+-
  Zero-Order Hold : ZeroOrderHold  SampleTime=-1
  upcoming speed (m/s) : Lookup_n-D  NumberOfTableDimensions=1  BreakpointsForDimension1=SegNo  BreakpointsForDimension2=G1Inprpm  Table=SegSPLatinmps  InterpMethod=Linear Lagrange  InternalRulePriority=Speed  RndMeth=Simplest  InputSameDT=on
  Dec_OR : Outport
  wires:
  Add3/1 -> upcoming speed (m/s)/1
  Ceil/1 -> Add3/1, SCP/1  "no interpolation done  as ceil values are used"
  SCP/1 -> Subtract/2
  Constant/1 -> Add3/2
  Subtract/1 -> If1/1, Scope/1  "Dist2SCP (m)"
  Segment number/1 -> Ceil/1
  Magnitude Squared/1 -> Subtract1/1
  Constant4/1 -> Gain2/1  "deceleration in m/s^2"
  Divide/1 -> Abs/1  "Dist2Dec (m)"
  Constant1/1 -> If Action Subsystem1/1(In1)
  Constant2/1 -> If Action Subsystem2/1(In1)
  If1/1 -> If Action Subsystem2/Action
  If Action Subsystem2/1(Out1) -> Merge/1
  Magnitude Squared1/1 -> Subtract1/2
  Merge/1 -> Data Type Conversion/1, Scope2/1
  Data Type Conversion/1 -> Dec_OR/1
  Max Speed Profile (m/s)/1 -> Magnitude Squared1/1
  d (m)/1 -> Subtract/1, Zero-Order Hold/1, Segment number/1  "Index distance for vehicle position"
  Subtract1/1 -> Divide/1
  Gain2/1 -> Gain/1
  Gain/1 -> Divide/2
  If1/2 -> If Action Subsystem1/Action
  Zero-Order Hold/1 -> Max Speed Profile (m/s)/1
  If Action Subsystem1/1(Out1) -> Merge/2
  v (m/s)/1 -> If1/4  "v (m/s)"
  upcoming speed (m/s)/1 -> If1/3, Magnitude Squared/1
  Abs/1 -> Gain1/1
  Gain1/1 -> Scope/2, If1/2

== system Refined_Model_38/Driver Model/Acc//Dec Control/Stop duration ==
  d (m) : Inport
  1-D Lookup Table : Lookup_n-D  NumberOfTableDimensions=1  BreakpointsForDimension1=Stoptimes(:,1)  Table=1:length(Stoptimes)  InternalRulePriority=Speed  RndMeth=Simplest  InputSameDT=on
  Ceil : Rounding  Operator=ceil
  Constant2 : Constant
  Direct Lookup Table (n-D) : LookupNDDirect  NumberOfTableDimensions=1  Table=Stoptimes(:,2)
  Scope : Scope
  Subtract1 : Sum  Inputs=+-
  Stop_t (s) : Outport
  wires:
  1-D Lookup Table/1 -> Ceil/1
  d (m)/1 -> 1-D Lookup Table/1
  Subtract1/1 -> Direct Lookup Table (n-D)/1
  Direct Lookup Table (n-D)/1 -> Stop_t (s)/1, Scope/1  "Stop time (s)"
  Ceil/1 -> Subtract1/1
  Constant2/1 -> Subtract1/2

== system Refined_Model_38/Driver Model/Acc//Dec Control/Trip complete ==
  d (m) : Inport
  Constant1 : Constant  Value=NoSteps
  Constant2 : Constant
  Delay : Delay  DelayLength=1
  Derivative : Derivative
  If : If  NumInputs=3  IfExpression=u1 > u2 & u3 ==0  ShowElse=off
  If Action Subsystem : Subsystem  TreatAsAtomicUnit=on
  Stop Simulation : Stop
  wires:
  Constant1/1 -> If/2
  Constant2/1 -> If Action Subsystem/1(In1)
  If/1 -> If Action Subsystem/Action
  If Action Subsystem/1(Out1) -> Delay/1
  d (m)/1 -> If/1, Derivative/1
  Delay/1 -> Stop Simulation/1
  Derivative/1 -> If/3  "v (m/s)"

== system Refined_Model_38/Driver Model/Driver Throttle/Idling// Apos = 0 ==
  Apos(m/s^2) : Inport
  Constant : Constant
  Constant2 : Constant  Value=0
  Idling : If  IfExpression=u1 == 0
  If Action Subsystem : Subsystem  TreatAsAtomicUnit=on
  If Action Subsystem1 : Subsystem  TreatAsAtomicUnit=on
  Merge : Merge
  Azero : Outport
  wires:
  Constant2/1 -> If Action Subsystem1/1(In1)
  Idling/1 -> If Action Subsystem/Action
  Merge/1 -> Azero/1
  If Action Subsystem1/1(Out1) -> Merge/1
  Constant/1 -> If Action Subsystem/1(In1)
  Apos(m/s^2)/1 -> Idling/1
  Idling/2 -> If Action Subsystem1/Action
  If Action Subsystem/1(Out1) -> Merge/2

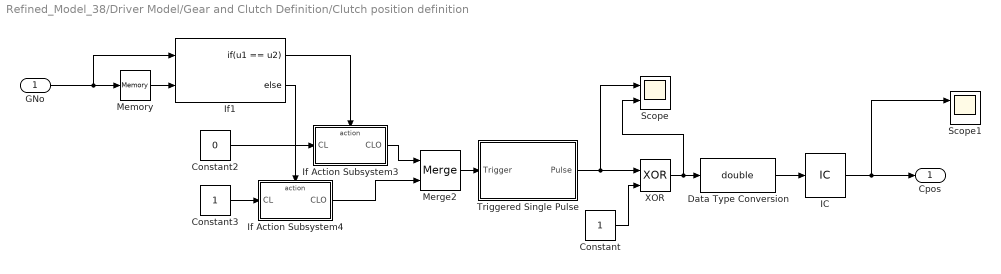
== system Refined_Model_38/Driver Model/Gear and Clutch Definition/Clutch position definition ==
  GNo : Inport
  Constant : Constant
  Constant2 : Constant  Value=0
  Constant3 : Constant
  Data Type Conversion : DataTypeConversion  OutDataTypeStr=double
  IC : InitialCondition  Value=0
  If Action Subsystem3 : Subsystem  TreatAsAtomicUnit=on
  If Action Subsystem4 : Subsystem  TreatAsAtomicUnit=on
  If1 : If  NumInputs=2  IfExpression=u1 == u2
  Memory : Memory
  Merge2 : Merge
  Scope : Scope  NumInputPorts=2
  Scope1 : Scope  NumInputPorts=2
  Triggered Single Pulse : Subsystem  TreatAsAtomicUnit=on  mask(single pulse generation){p_wid=10}
      mask prompts: p_wid "pulse width (number of samples)"
      mask help: This block generate a single pulse whenever a trigger happen. The pulse width must specified as a number of samples. for example if your sampling time is 0.1s and you want 3s pulse , then you should enter 30 as a pulse width.
      mask Display:
      | plot([0],[0])
      | plot([11],[0])
      | plot([5],[0.5])
      | plot([4 5 5 6 6 7],[0 0 0.25 0.25 0 0])
      | plot([5],[-0.3])
      | 
      | port_label('output', 1, 'Pulse')
      | port_label('input', 1, 'Trigger')
  XOR : Logic  Operator=XOR  IconShape=distinctive  AllPortsSameDT=off  OutDataTypeStr=boolean
  Cpos : Outport
  wires:
  If1/1 -> If Action Subsystem3/Action
  If Action Subsystem3/1(CLO) -> Merge2/1
  Memory/1 -> If1/2
  Constant2/1 -> If Action Subsystem3/1(CL)
  Constant3/1 -> If Action Subsystem4/1(CL)
  GNo/1 -> Memory/1, If1/1
  If1/2 -> If Action Subsystem4/Action
  If Action Subsystem4/1(CLO) -> Merge2/2
  Merge2/1 -> Triggered Single Pulse/1(Trigger)
  Triggered Single Pulse/1(Pulse) -> Scope/1, XOR/1
  Constant/1 -> XOR/2
  XOR/1 -> Scope/2, Data Type Conversion/1
  Data Type Conversion/1 -> IC/1
  IC/1 -> Cpos/1, Scope1/1

== system Refined_Model_38/Driver Model/Gear and Clutch Definition/If Action Subsystem3 ==
  Selected Gear /dt : Inport
  Action Port : ActionPort  ActionPortLabel=if(u1 >= u2)
  Add : Sum
  Constant : Constant
  Increased gear : Outport
  wires:
  Selected Gear /dt/1 -> Add/1
  Add/1 -> Increased gear/1
  Constant/1 -> Add/2

== system Refined_Model_38/Driver Model/Gear and Clutch Definition/If Action Subsystem4 ==
  Selected Gear /dt : Inport
  Action Port : ActionPort  ActionPortLabel=elseif(u3 >= u4)
  Constant : Constant
  Subtract : Sum  Inputs=+-
  Decreased gear : Outport
  wires:
  Constant/1 -> Subtract/2
  Subtract/1 -> Decreased gear/1
  Selected Gear /dt/1 -> Subtract/1

== system Refined_Model_38/Driver Model/Gear and Clutch Definition/If Action Subsystem5 ==
  Selected Gear Ratio /dt : Inport
  Action Port : ActionPort  ActionPortLabel=else
  Out1 : Outport
  wires:
  Selected Gear Ratio /dt/1 -> Out1/1

== system Refined_Model_38/Driver Model/Gear and Clutch Definition/If Action Subsystem6 ==
  In1 : Inport
  Action Port : ActionPort  ActionPortLabel=elseif(u1 == 0)
  Out1 : Outport
  wires:
  In1/1 -> Out1/1

== system Refined_Model_38/Vehicle Model/Engine Model/Clutch ==
  Cpos : Inport
  T_e (Nm) : Inport  Port=2
  T_e_inertia (Nm) : Inport  Port=3
  Clutch value1 : Product
  Gain20 : Gain  Gain=etaClutch
  IC2 : InitialCondition  Value=0
  Saturation2 : Saturate  UpperLimit=inf  LowerLimit=0
  Scope : Scope
  Scope1 : Scope  NumInputPorts=2
  Subtract : Sum  Inputs=+-
  T_c (Nm) : Outport
  wires:
  IC2/1 -> Clutch value1/1
  Clutch value1/1 -> Scope1/1, Subtract/1
  Cpos/1 -> IC2/1
  Gain20/1 -> Saturation2/1  "T_c (Nm)"
  T_e_inertia (Nm)/1 -> Scope1/2, Subtract/2
  T_e (Nm)/1 -> Clutch value1/2
  Saturation2/1 -> Scope/1, T_c (Nm)/1
  Subtract/1 -> Gain20/1

== system Refined_Model_38/Driver Model/Acc//Dec Control/Idling state/If Action Subsystem ==
  In1 : Inport
  Action Port : ActionPort  ActionPortLabel=if(u1 == 0 & u2 < 0 & u3 > 10)
  Out1 : Outport
  wires:
  In1/1 -> Out1/1

== system Refined_Model_38/Driver Model/Acc//Dec Control/Idling state/If Action Subsystem1 ==
  In1 : Inport
  Action Port : ActionPort  ActionPortLabel=else
  Out1 : Outport
  wires:
  In1/1 -> Out1/1

== system Refined_Model_38/Driver Model/Acc//Dec Control/Look Ahead Braking Model/If Action Subsystem1 ==
  In1 : Inport
  Action Port : ActionPort  ActionPortLabel=else
  Out1 : Outport
  wires:
  In1/1 -> Out1/1

== system Refined_Model_38/Driver Model/Acc//Dec Control/Look Ahead Braking Model/If Action Subsystem2 ==
  In1 : Inport
  Action Port : ActionPort  ActionPortLabel=if(u1 <= u2 & u4 > u3)
  Out1 : Outport
  wires:
  In1/1 -> Out1/1

== system Refined_Model_38/Driver Model/Acc//Dec Control/Trip complete/If Action Subsystem ==
  In1 : Inport
  Action Port : ActionPort  ActionPortLabel=if(u1 > u2 & u3 ==0)
  Out1 : Outport
  wires:
  In1/1 -> Out1/1

== system Refined_Model_38/Driver Model/Driver Throttle/Idling// Apos = 0/If Action Subsystem ==
  In1 : Inport
  Action Port : ActionPort  ActionPortLabel=if(u1 == 0)
  Out1 : Outport
  wires:
  In1/1 -> Out1/1

== system Refined_Model_38/Driver Model/Driver Throttle/Idling// Apos = 0/If Action Subsystem1 ==
  In1 : Inport
  Action Port : ActionPort  ActionPortLabel=else
  Out1 : Outport
  wires:
  In1/1 -> Out1/1

== system Refined_Model_38/Driver Model/Gear and Clutch Definition/Clutch position definition/If Action Subsystem3 ==
  CL : Inport
  Action Port : ActionPort  ActionPortLabel=if(u1 == u2)
  CLO : Outport
  wires:
  CL/1 -> CLO/1

== system Refined_Model_38/Driver Model/Gear and Clutch Definition/Clutch position definition/If Action Subsystem4 ==
  CL : Inport
  Action Port : ActionPort  ActionPortLabel=else
  CLO : Outport
  wires:
  CL/1 -> CLO/1

== system Refined_Model_38/Driver Model/Gear and Clutch Definition/Clutch position definition/Triggered Single Pulse ==
  Trigger : Inport
  +ve edge detect : Subsystem
  Add : Sum
  Add1 : Sum
  Compare To Constant : simulink/Logic and Bit Operations/Compare To Constant  relop=>  const=p_wid-1  OutDataTypeStr=boolean
  Constant2 : Constant
  Logical Operator : Logic  Operator=NOT  AllPortsSameDT=off  OutDataTypeStr=boolean
  Product : Product  RndMeth=Zero
  Product1 : Product  RndMeth=Zero
  Product3 : Product  RndMeth=Zero
  Saturation : Saturate  UpperLimit=1  LowerLimit=0
  Unit Delay : UnitDelay  SampleTime=-1  HasFrameUpgradeWarning=on
  Unit Delay1 : UnitDelay  SampleTime=-1  HasFrameUpgradeWarning=on
  Pulse : Outport
  wires:
  Compare To Constant/1 -> Logical Operator/1
  Constant2/1 -> Product/1
  Product/1 -> Add/1
  Unit Delay/1 -> Add/2, Compare To Constant/1
  Trigger/1 -> +ve edge detect/1(signal)
  +ve edge detect/1(out) -> Add1/2
  Add/1 -> Product1/2
  Product1/1 -> Unit Delay/1
  Add1/1 -> Unit Delay1/1
  Unit Delay1/1 -> Saturation/1
  Saturation/1 -> Product3/1
  Product3/1 -> Add1/1, Product/2, Product1/1, Pulse/1
  Logical Operator/1 -> Product3/2

== system Refined_Model_38/Driver Model/Gear and Clutch Definition/Clutch position definition/Triggered Single Pulse/+ve edge detect ==
  note: Edge
  signal : Inport
  Delay Input1 : UnitDelay  Description=Store in Global RAM  DisableCoverage=on  SampleTime=-1  HasFrameUpgradeWarning=on
  FixPt Relational Operator : RelationalOperator  Operator=>  OutDataTypeStr=fixdt(0, 8)  ZeroCross=off  RndMeth=Nearest
  Positive : simulink/Logic and Bit Operations/Compare To Zero  relop=>  OutDataTypeStr=uint8  ZeroCross=off
  out : Outport
  wires:
  Delay Input1/1 -> FixPt Relational Operator/2  "U(k-1)"
  Positive/1 -> Delay Input1/1, FixPt Relational Operator/1  "U(k)"
  FixPt Relational Operator/1 -> out/1
  signal/1 -> Positive/1
